simulink model "CART"  (R2024b)
settings: Solver=VariableStepAuto  StartTime=0.0  StopTime=10.0  RelTol=1e-3
settings Model: Creator=quinn  LastModifiedBy=quinn

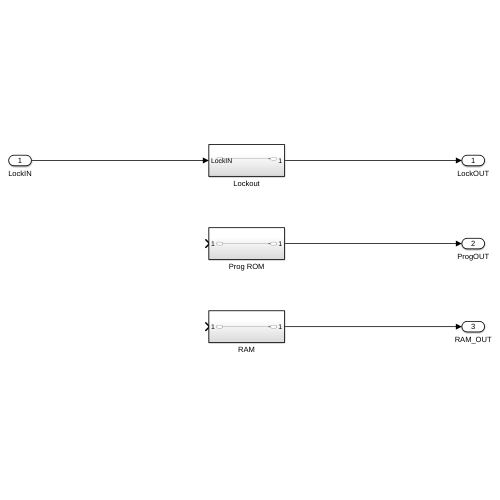
[thumbnail: Simulink's stored preview of the top-level diagram]
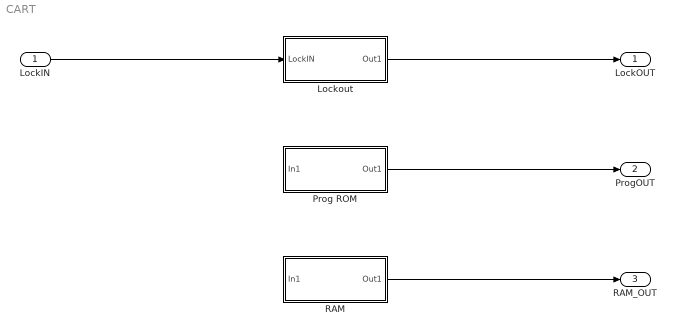
== system CART ==
  LockIN : Inport
  Lockout : Subsystem
  Prog ROM : Subsystem
  RAM : Subsystem
  LockOUT : Outport
  ProgOUT : Outport  Port=2
  RAM_OUT : Outport  Port=3
  wires:
  Lockout/1(Out1) -> LockOUT/1
  Prog ROM/1(Out1) -> ProgOUT/1
  RAM/1(Out1) -> RAM_OUT/1
  LockIN/1 -> Lockout/1(LockIN)

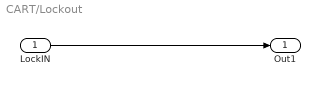
== system CART/Lockout ==
  LockIN : Inport
  Out1 : Outport
  wires:
  LockIN/1 -> Out1/1

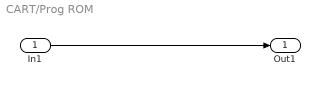
== system CART/Prog ROM ==
  In1 : Inport
  Out1 : Outport
  wires:
  In1/1 -> Out1/1

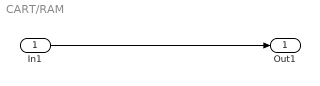
== system CART/RAM ==
  In1 : Inport
  Out1 : Outport
  wires:
  In1/1 -> Out1/1
